simulink model "Steps_HW_2025"  (R2024b)
settings: Solver=FixedStepDiscrete  StartTime=0.0  StopTime=inf  RelTol=1e-3
libraries: microbitledlib x15, simulink x10, microbitaccellib x2, microbitbuttonlib x1
settings Model: ExtModeTrigDuration=5  Creator=eelkhour  LastModifiedBy=ahenshaw
settings OptimizationCC: EnhancedBackFolding=on  PassReuseOutputArgsAs=Individual arguments  ZeroExternalMemoryAtStartup=off  ZeroInternalMemoryAtStartup=off  MaxStackSize=64  OptimizeBlockOrder=speed  DifferentSizesBufferReuse=on  OptimizationCustomize=off  EfficientTunableParamExpr=on
settings DebuggingCC: ParameterOverflowMsg=none  ParameterTunabilityLossMsg=error
settings HardwareCC: ProdBitPerPointer=32  ProdBitPerSizeT=32  ProdBitPerPtrDiffT=32  ProdLargestAtomicInteger=Long  ProdLargestAtomicFloat=Double  ProdWordSize=32  ProdHWDeviceType=ARM Compatible->ARM Cortex
settings SFSimCC: MATLABDynamicMemAlloc=off
settings RTWCC: Description=Embedded Coder  SystemTargetFile=ert.tlc  HardwareBoard=BBC micro:bit V2  TemplateMakefile=ert_default_tmf  Toolchain=GNU Tools for ARM Embedded Processors  GPUComputeCapability=3.5
settings CodeAppCC: ForceParamTrailComments=on  IgnoreCustomStorageClasses=off  OperatorAnnotations=on  SimulinkDataObjDesc=on  SFDataObjDesc=on  InsertBlockDesc=on
settings ERTTargetCC: ExtModeTransport=3  ExtModeStaticAlloc=on  ExtModeMexFile=ext_xcp  ExtModeIntrfLevel=Level2 - Open  InlinedParameterPlacement=Hierarchical  DynamicArrayContainerType=coder::array

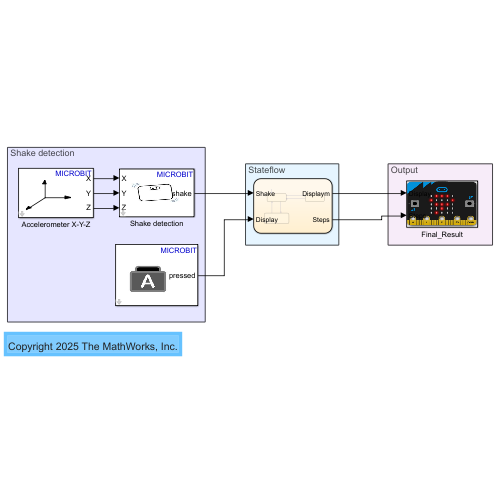
[thumbnail: Simulink's stored preview of the top-level diagram]
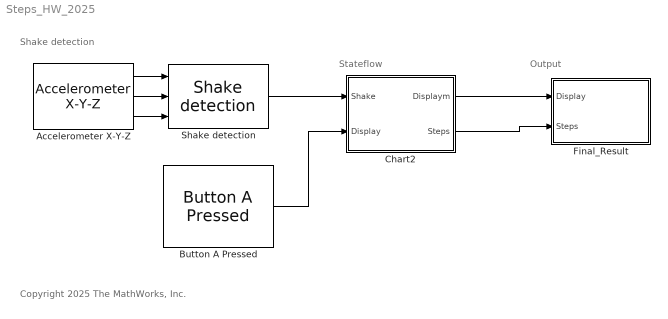
== system Steps_HW_2025 ==
  note: Shake detection
  note: Stateflow
  note: Output
  note: Copyright 2025 The MathWorks, Inc.
  Accelerometer X-Y-Z : microbitaccellib/Accelerometer X-Y-Z  ODR=50Hz  Accelfullrange=-8g to +8g  SampleTime=0.1
  Button A Pressed : microbitbuttonlib/Button A Pressed  SampleTime=0.1
  Chart2 : Stateflow chart  TreatAsAtomicUnit=on
  Final_Result : Subsystem
      mask Display: image('Capture.PNG');
  Shake detection : microbitaccellib/Shake detection  sen=3
  wires:
  Accelerometer X-Y-Z/2 -> Shake detection/2
  Shake detection/1 -> Chart2/1(Shake)
  Accelerometer X-Y-Z/1 -> Shake detection/1
  Button A Pressed/1 -> Chart2/2(Display)
  Accelerometer X-Y-Z/3 -> Shake detection/3
  Chart2/2(Steps) -> Final_Result/2(Steps)
  Chart2/1(Displaym) -> Final_Result/1(Display)

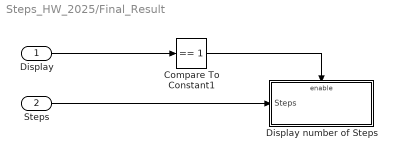
== system Steps_HW_2025/Final_Result ==
  Display : Inport
  Steps : Inport  Port=2
  Compare To Constant1 : simulink/Logic and Bit Operations/Compare To Constant  relop===  const=1  OutDataTypeStr=boolean
  Display number of Steps : Subsystem  TreatAsAtomicUnit=on
  wires:
  Compare To Constant1/1 -> Display number of Steps/Enable
  Steps/1 -> Display number of Steps/1(Steps)
  Display/1 -> Compare To Constant1/1

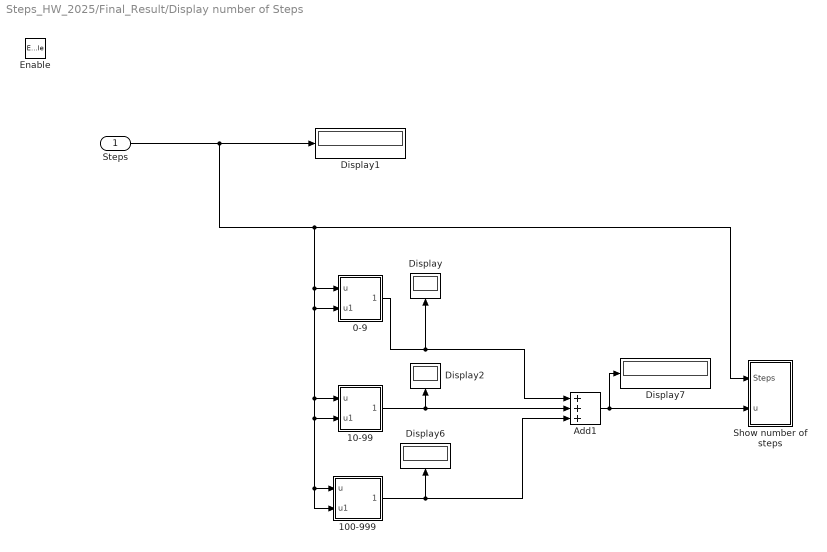
== system Steps_HW_2025/Final_Result/Display number of Steps ==
  Steps : Inport
  Enable : EnablePort
  0-9 : Subsystem
  10-99 : Subsystem
  100-999 : Subsystem
  Add1 : Sum  Inputs=+++
  Display{,1..2,6..7} (5 alike) : Display
  Show number of steps : Subsystem
  wires:
  100-999/1(Out1) -> Add1/3, Display6/1
  10-99/1(Out1) -> Display2/1, Add1/2
  Steps/1 -> Show number of steps/1(Steps), 100-999/2(u1), 100-999/1(u), 10-99/2(u1), 10-99/1(u), 0-9/2(u1), 0-9/1(u), Display1/1
  0-9/1(Out1) -> Add1/1, Display/1
  Add1/1 -> Show number of steps/2(u), Display7/1

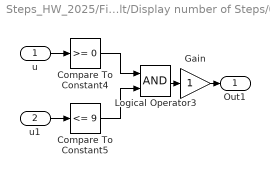
== system Steps_HW_2025/Final_Result/Display number of Steps/0-9 ==
  u : Inport
  u1 : Inport  Port=2
  Compare To Constant4 : simulink/Logic and Bit Operations/Compare To Constant  relop=>=  const=0  OutDataTypeStr=boolean
  Compare To Constant5 : simulink/Logic and Bit Operations/Compare To Constant  relop=<=  const=9  OutDataTypeStr=boolean
  Gain : Gain
  Logical Operator3 : Logic  AllPortsSameDT=off  OutDataTypeStr=boolean
  Out1 : Outport
  wires:
  Compare To Constant4/1 -> Logical Operator3/1
  Compare To Constant5/1 -> Logical Operator3/2
  u/1 -> Compare To Constant4/1
  u1/1 -> Compare To Constant5/1
  Logical Operator3/1 -> Gain/1
  Gain/1 -> Out1/1

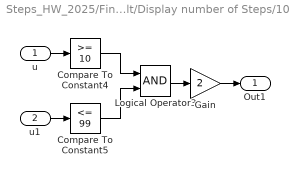
== system Steps_HW_2025/Final_Result/Display number of Steps/10-99 ==
  u : Inport
  u1 : Inport  Port=2
  Compare To Constant4 : simulink/Logic and Bit Operations/Compare To Constant  relop=>=  const=10  OutDataTypeStr=boolean
  Compare To Constant5 : simulink/Logic and Bit Operations/Compare To Constant  relop=<=  const=99  OutDataTypeStr=boolean
  Gain : Gain  Gain=2
  Logical Operator3 : Logic  AllPortsSameDT=off  OutDataTypeStr=boolean
  Out1 : Outport
  wires:
  u1/1 -> Compare To Constant5/1
  u/1 -> Compare To Constant4/1
  Compare To Constant5/1 -> Logical Operator3/2
  Compare To Constant4/1 -> Logical Operator3/1
  Logical Operator3/1 -> Gain/1
  Gain/1 -> Out1/1

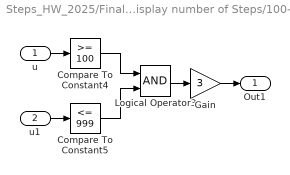
== system Steps_HW_2025/Final_Result/Display number of Steps/100-999 ==
  u : Inport
  u1 : Inport  Port=2
  Compare To Constant4 : simulink/Logic and Bit Operations/Compare To Constant  relop=>=  const=100  OutDataTypeStr=boolean
  Compare To Constant5 : simulink/Logic and Bit Operations/Compare To Constant  relop=<=  const=999  OutDataTypeStr=boolean
  Gain : Gain  Gain=3
  Logical Operator3 : Logic  AllPortsSameDT=off  OutDataTypeStr=boolean
  Out1 : Outport
  wires:
  Compare To Constant4/1 -> Logical Operator3/1
  Compare To Constant5/1 -> Logical Operator3/2
  u/1 -> Compare To Constant4/1
  u1/1 -> Compare To Constant5/1
  Logical Operator3/1 -> Gain/1
  Gain/1 -> Out1/1

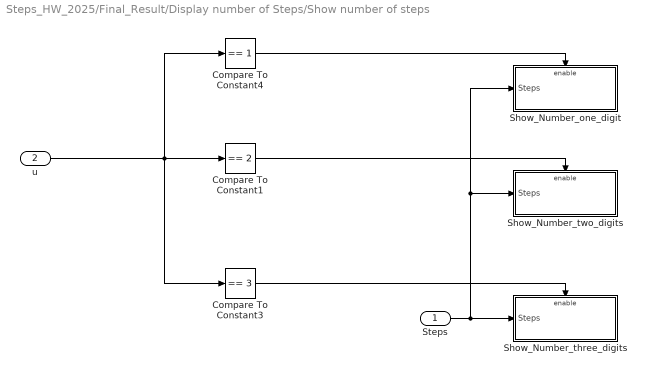
== system Steps_HW_2025/Final_Result/Display number of Steps/Show number of steps ==
  Steps : Inport
  u : Inport  Port=2
  Compare To Constant1 : simulink/Logic and Bit Operations/Compare To Constant  relop===  const=2  OutDataTypeStr=boolean
  Compare To Constant3 : simulink/Logic and Bit Operations/Compare To Constant  relop===  const=3  OutDataTypeStr=boolean
  Compare To Constant4 : simulink/Logic and Bit Operations/Compare To Constant  relop===  const=1  OutDataTypeStr=boolean
  Show_Number_one_digit : Subsystem  TreatAsAtomicUnit=on
  Show_Number_three_digits : Subsystem  TreatAsAtomicUnit=on
  Show_Number_two_digits : Subsystem  TreatAsAtomicUnit=on
  wires:
  Compare To Constant1/1 -> Show_Number_two_digits/Enable
  Compare To Constant3/1 -> Show_Number_three_digits/Enable
  Steps/1 -> Show_Number_one_digit/1(Steps), Show_Number_two_digits/1(Steps), Show_Number_three_digits/1(Steps)
  u/1 -> Compare To Constant4/1, Compare To Constant3/1, Compare To Constant1/1
  Compare To Constant4/1 -> Show_Number_one_digit/Enable

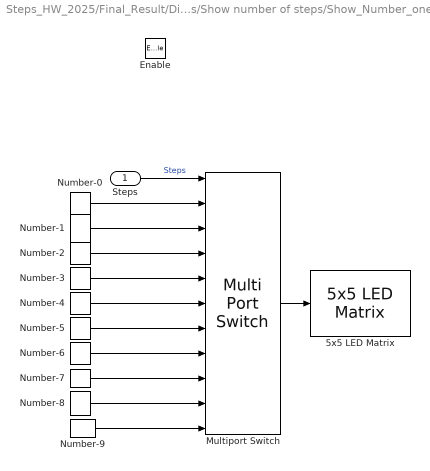
== system Steps_HW_2025/Final_Result/Display number of Steps/Show number of steps/Show_Number_one_digit ==
  Steps : Inport
  Enable : EnablePort
  5x5 LED Matrix : microbitledlib/5x5 LED Matrix  LED_mat=[0 1 1 1 0;1 0 1 0 1;1 1 0 1 1; 1 0 1 0 1;0 1 1 1 0]
  Multiport Switch : MultiPortSwitch  DataPortOrder=Specify indices  Inputs=9  DataPortIndices={0,1,2,3,4,5,6,7,8,9}  DiagnosticForDefault=None  SaturateOnIntegerOverflow=off  InputSameDT=off
  Number-0 : microbitledlib/LED Images/Number-0  L00=off  L01=on  L02=on  L03=off  L04=off  L10=on  L11=off  L12=off  L13=on  L14=off  L20=on  L21=off  L22=off  L23=on  L24=off  L30=on  L31=off  L32=off  L33=on  L34=off  L40=off  L41=on  L42=on  L43=off  L44=off
  Number-1 : microbitledlib/LED Images/Number-1  L00=off  L01=off  L02=on  L03=off  L04=off  L10=off  L11=on  L12=on  L13=off  L14=off  L20=off  L21=off  L22=on  L23=off  L24=off  L30=off  L31=off  L32=on  L33=off  L34=off  L40=off  L41=on  L42=on  L43=on  L44=off
  Number-2 : microbitledlib/LED Images/Number-2  L00=on  L01=on  L02=on  L03=off  L04=off  L10=off  L11=off  L12=off  L13=on  L14=off  L20=off  L21=on  L22=on  L23=on  L24=off  L30=on  L31=off  L32=off  L33=off  L34=off  L40=on  L41=on  L42=on  L43=on  L44=off
  Number-3 : microbitledlib/LED Images/Number-3  L00=on  L01=on  L02=on  L03=on  L04=off  L10=off  L11=off  L12=off  L13=on  L14=off  L20=off  L21=off  L22=on  L23=off  L24=off  L30=on  L31=off  L32=off  L33=on  L34=off  L40=off  L41=on  L42=on  L43=off  L44=off
  Number-4 : microbitledlib/LED Images/Number-4  L00=off  L01=off  L02=on  L03=on  L04=off  L10=off  L11=on  L12=off  L13=on  L14=off  L20=on  L21=off  L22=off  L23=on  L24=off  L30=on  L31=on  L32=on  L33=on  L34=on  L40=off  L41=off  L42=off  L43=on  L44=off
  Number-5 : microbitledlib/LED Images/Number-5  L00=on  L01=on  L02=on  L03=on  L04=on  L10=on  L11=off  L12=off  L13=off  L14=off  L20=on  L21=on  L22=on  L23=on  L24=off  L30=off  L31=off  L32=off  L33=off  L34=on  L40=on  L41=on  L42=on  L43=on  L44=off
  Number-6 : microbitledlib/LED Images/Number-6  L00=off  L01=off  L02=off  L03=on  L04=off  L10=off  L11=off  L12=on  L13=off  L14=off  L20=off  L21=on  L22=on  L23=on  L24=off  L30=on  L31=off  L32=off  L33=off  L34=on  L40=off  L41=on  L42=on  L43=on  L44=off
  Number-7 : microbitledlib/LED Images/Number-7  L00=on  L01=on  L02=on  L03=on  L04=on  L10=off  L11=off  L12=off  L13=on  L14=off  L20=off  L21=off  L22=on  L23=off  L24=off  L30=off  L31=on  L32=off  L33=off  L34=off  L40=on  L41=off  L42=off  L43=off  L44=off
  Number-8 : microbitledlib/LED Images/Number-8  L00=off  L01=on  L02=on  L03=on  L04=off  L10=on  L11=off  L12=off  L13=off  L14=on  L20=off  L21=on  L22=on  L23=on  L24=off  L30=on  L31=off  L32=off  L33=off  L34=on  L40=off  L41=on  L42=on  L43=on  L44=off
  Number-9 : microbitledlib/LED Images/Number-9  L00=off  L01=on  L02=on  L03=on  L04=off  L10=on  L11=off  L12=off  L13=off  L14=on  L20=off  L21=on  L22=on  L23=on  L24=off  L30=off  L31=off  L32=on  L33=off  L34=off  L40=off  L41=on  L42=off  L43=off  L44=off
  wires:
  Number-6/1 -> Multiport Switch/8
  Number-5/1 -> Multiport Switch/7
  Number-2/1 -> Multiport Switch/4
  Multiport Switch/1 -> 5x5 LED Matrix/1
  Number-4/1 -> Multiport Switch/6
  Number-1/1 -> Multiport Switch/3
  Number-7/1 -> Multiport Switch/9
  Number-3/1 -> Multiport Switch/5
  Steps/1 -> Multiport Switch/1  "Steps"
  Number-8/1 -> Multiport Switch/10
  Number-9/1 -> Multiport Switch/11
  Number-0/1 -> Multiport Switch/2

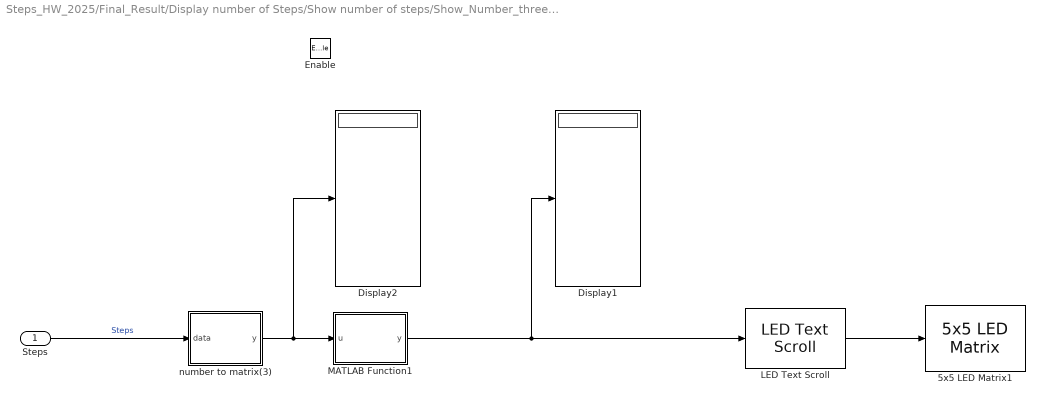
== system Steps_HW_2025/Final_Result/Display number of Steps/Show number of steps/Show_Number_three_digits ==
  Steps : Inport
  Enable : EnablePort
  5x5 LED Matrix1 : microbitledlib/5x5 LED Matrix  LED_mat=[0 1 1 1 0;1 0 1 0 1;1 1 0 1 1; 1 0 1 0 1;0 1 1 1 0]
  Display1 : Display
  Display2 : Display
  LED Text Scroll : microbitledlib/LED Text Scroll  Speed=5
  MATLAB Function1 : MATLAB Function  TreatAsAtomicUnit=on
  number to matrix(3) : MATLAB Function  TreatAsAtomicUnit=on
  wires:
  MATLAB Function1/1(y) -> LED Text Scroll/1, Display1/1
  LED Text Scroll/1 -> 5x5 LED Matrix1/1
  number to matrix(3)/1(y) -> Display2/1, MATLAB Function1/1(u)
  Steps/1 -> number to matrix(3)/1(data)  "Steps"

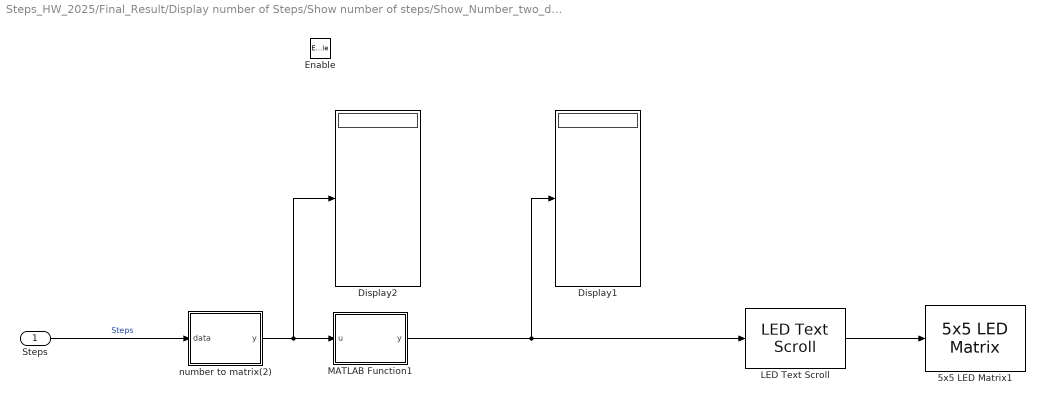
== system Steps_HW_2025/Final_Result/Display number of Steps/Show number of steps/Show_Number_two_digits ==
  Steps : Inport
  Enable : EnablePort
  5x5 LED Matrix1 : microbitledlib/5x5 LED Matrix  LED_mat=[0 1 1 1 0;1 0 1 0 1;1 1 0 1 1; 1 0 1 0 1;0 1 1 1 0]
  Display1 : Display
  Display2 : Display
  LED Text Scroll : microbitledlib/LED Text Scroll  Speed=5
  MATLAB Function1 : MATLAB Function  TreatAsAtomicUnit=on
  number to matrix(2) : MATLAB Function  TreatAsAtomicUnit=on
  wires:
  MATLAB Function1/1(y) -> LED Text Scroll/1, Display1/1
  LED Text Scroll/1 -> 5x5 LED Matrix1/1
  number to matrix(2)/1(y) -> Display2/1, MATLAB Function1/1(u)
  Steps/1 -> number to matrix(2)/1(data)  "Steps"

== stateflow chart Steps_HW_2025/Chart2 ==
  state Not_shaking
    entry:
    Displaym=  0;
  state Shaking
    entry:
    Steps = Steps +1;
  state Display_Steps
    entry:
    Displaym=  1;
  (default) -> Not_shaking
  Not_shaking -> Shaking [order 1] : [Shake== 1 ]
  Shaking -> Not_shaking : after(1,sec)
  Display_Steps -> Not_shaking : after(4,sec)
  Not_shaking -> Display_Steps [order 2] : [Display== 1 ]
  data: Shake input; Display input; Displaym output; Steps output =0

== matlab function Steps_HW_2025/Final_Result/Display number of Steps/Show number of steps/Show_Number_two_digits/number to matrix(2) ==
  data: y output; data input
function y = fcn(data)


    c=zeros(1,2);
    c(1,1)=mod(data,10)+48;
    data=floor(data/10);
    c(1,2)=mod(data,10)+48;
    c=flip(c);
    y=c;

== matlab function Steps_HW_2025/Final_Result/Display number of Steps/Show number of steps/Show_Number_two_digits/MATLAB Function1 ==
  data: y output; u input
function y = fcn(u)


if(size(u,1)>1) % do this check for constant blocks, where the
    uu = u';
else
    uu=u;
end

uu=upper(char(uu));

y = uint8(horzcat(uint8(uu) , zeros(1 , 254 - size(uu, 2))));

== matlab function Steps_HW_2025/Final_Result/Display number of Steps/Show number of steps/Show_Number_three_digits/MATLAB Function1 ==
  data: y output; u input
function y = fcn(u)


if(size(u,1)>1) % do this check for constant blocks, where the
    uu = u';
else
    uu=u;
end

uu=upper(char(uu));

y = uint8(horzcat(uint8(uu) , zeros(1 , 254 - size(uu, 2))));

== matlab function Steps_HW_2025/Final_Result/Display number of Steps/Show number of steps/Show_Number_three_digits/number to matrix(3) ==
  data: y output; data input
function y = fcn(data)


    c=zeros(1,3);
    c(1,1)=mod(data,10)+48;

    data=floor(data/10);
    c(1,2)=mod(data,10)+48;

    data=floor(data/10);
    c(1,3)=mod(data,10)+48;

    c=flip(c);
    y=c;
